simulink model "implementacion_ec_diferencia"  (R2020b)
settings: Solver=VariableStepAuto  StartTime=0.0  StopTime=10.0  RelTol=1e-3
values from neighbouring files (symbols this model uses):
  Tm = 0.01    [control_algebraico_dig.m]    (also in control_digital.m)
settings Model: Creator=Acer  LastModifiedBy=Acer

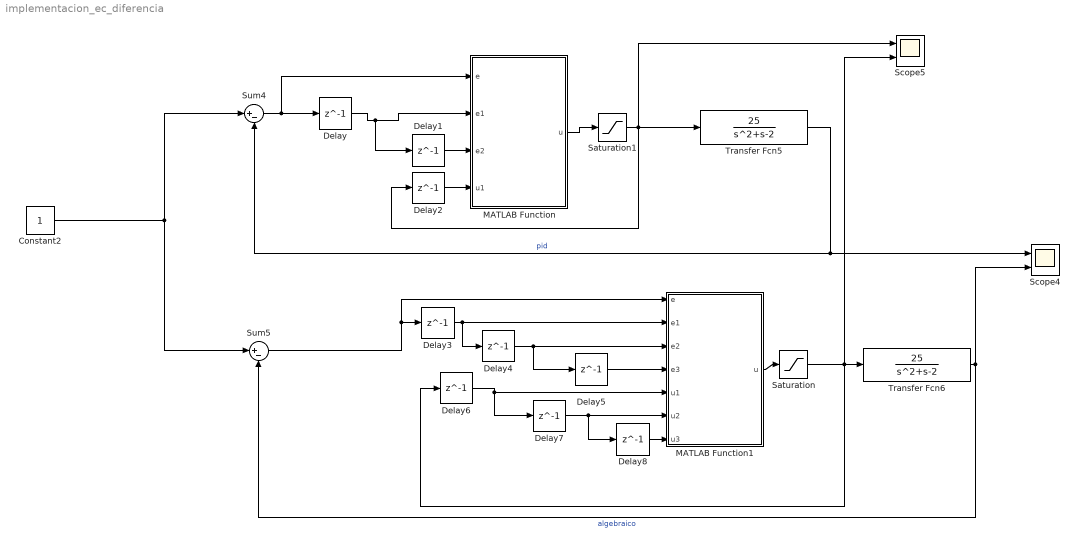
== system implementacion_ec_diferencia ==
  Constant2 : Constant
  Delay{,1..8} (9 alike) : Delay  DelayLength=1  SampleTime=Tm
  MATLAB Function : MATLAB Function  TreatAsAtomicUnit=on
  MATLAB Function1 : MATLAB Function  TreatAsAtomicUnit=on
  Saturation : Saturate  UpperLimit=10  LowerLimit=-10
  Saturation1 : Saturate  UpperLimit=10  LowerLimit=-10
  Scope4 : Scope  NumInputPorts=2
  Scope5 : Scope  NumInputPorts=2
  Sum4 : Sum  Inputs=|+-
  Sum5 : Sum  Inputs=|+-
  Transfer Fcn5 : TransferFcn  Numerator=[25]  Denominator=[1 1 -2]
  Transfer Fcn6 : TransferFcn  Numerator=[25]  Denominator=[1 1 -2]
  wires:
  MATLAB Function/1(u) -> Saturation1/1
  Sum5/1 -> Delay3/1, MATLAB Function1/1(e)
  Constant2/1 -> Sum5/1, Sum4/1
  MATLAB Function1/1(u) -> Saturation/1
  Transfer Fcn5/1 -> Scope4/1, Sum4/2  "pid"
  Transfer Fcn6/1 -> Scope4/2, Sum5/2  "algebraico"
  Saturation/1 -> Delay6/1, Scope5/2, Transfer Fcn6/1
  Delay/1 -> Delay1/1, MATLAB Function/2(e1)
  Delay1/1 -> MATLAB Function/3(e2)
  Delay2/1 -> MATLAB Function/4(u1)
  Delay3/1 -> Delay4/1, MATLAB Function1/2(e1)
  Delay4/1 -> Delay5/1, MATLAB Function1/3(e2)
  Delay5/1 -> MATLAB Function1/4(e3)
  Delay6/1 -> MATLAB Function1/5(u1), Delay7/1
  Delay7/1 -> Delay8/1, MATLAB Function1/6(u2)
  Delay8/1 -> MATLAB Function1/7(u3)
  Saturation1/1 -> Delay2/1, Scope5/1, Transfer Fcn5/1
  Sum4/1 -> MATLAB Function/1(e), Delay/1

== matlab function implementacion_ec_diferencia/MATLAB Function1 ==
  data: e input; u output; e1 input; e2 input; e3 input; u1 input; u2 input; u3 input
function u = fcn(e,e1,e2,e3,u1,u2,u3)
%e(k)--->e
%e(k-1)---> e1
%e(k-2)-->e2
%u(k-2)---> u2
u=1.268*e1- 2.492*e2+ 1.225*e3+2.629*u1-2.306*u2+0.6771*u3;

== matlab function implementacion_ec_diferencia/MATLAB Function ==
  data: e input; u output; e1 input; e2 input; u1 input
function u = fcn(e,e1,e2,u1)
%e(k)--->e
%e(k-1)---> e1
%e(k-2)-->e2
%u(k-2)---> u2
%u=160.5*e-312*e1+151.5*e2+u2;
Kp=4.4800;
Ti=2.24;
Td=0.1741;
T=0.01;
u= Kp*(e-e1+(Td/T)*(e-2*e1+e2)+(T/Ti)*e)+u1;
